simulink model "loader_est"  (R2025b)
settings: Solver=FixedStepAuto  StartTime=0.0  StopTime=26  FixedStep=0.001  RelTol=1e-3
undefined symbols (not defined in the file or in its folder): m_arm, m_bucket, m_load, X, Y, Z
libraries: sm_lib x31, nesl_utility x10, simulink x1
(part 2 of 2)

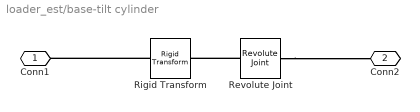
== system loader_est/base-tilt cylinder ==
  Revolute Joint : sm_lib/Joints/Revolute Joint  JointMode=Normal  CompositeWrenchDir=FollowerOnBase  CompositeWrenchFrame=BaseFrame  SenseConstraintForce=off  SenseConstraintTorque=off  SenseTotalForce=off  SenseTotalTorque=off  PositionTargetSpecify=off  PositionTargetPriority=High  PositionTargetValue=0  PositionTargetValueUnits=deg  VelocityTargetSpecify=off  VelocityTargetPriority=High  VelocityTargetValue=0  VelocityTargetValueUnits=deg/s  EquilibriumPosition=0  EquilibriumPositionUnits=deg  SpringStiffness=0  SpringStiffnessUnits=N*m/deg  DampingCoefficient=0  DampingCoefficientUnits=N*m/(deg/s)  LowerLimitSpecify=off  LowerLimitBound=-90  LowerLimitBoundUnits=deg  LowerLimitStiffness=1e4  LowerLimitStiffnessUnits=N*m/deg  LowerLimitDamping=10  LowerLimitDampingUnits=N*m/(deg/s)  LowerLimitTransitionRegionWidth=0.1  LowerLimitTransitionRegionWidthUnits=deg  UpperLimitSpecify=off  UpperLimitBound=90  UpperLimitBoundUnits=deg  UpperLimitStiffness=1e4  UpperLimitStiffnessUnits=N*m/deg  UpperLimitDamping=10  UpperLimitDampingUnits=N*m/(deg/s)  UpperLimitTransitionRegionWidth=0.1  UpperLimitTransitionRegionWidthUnits=deg  TorqueActuationMode=NoTorque  MotionActuationMode=ComputedMotion  SensePosition=off  SenseVelocity=off  SenseAcceleration=off  SenseTorqueForce=off  SenseLowerLimitTorqueForce=off  SenseUpperLimitTorqueForce=off
  Rigid Transform : sm_lib/Frames and Transforms/Rigid Transform  RotationMethod=RotationSequence  FollAlignAxisA=+X  BaseAlignAxisA=+Y  FollAlignAxisB=+Y  BaseAlignAxisB=+Z  RotationStandardAxis=+Z  RotationAngle=0  RotationAngleUnits=deg  RotationArbitraryAxis=[0 0 1]  RotationSequenceAxes=FollowerAxes  RotationSequence=XYX  RotationSequenceAngles=[90 180 0]  RotationSequenceAnglesUnits=deg  RotationMatrix=[1 0 0;0 1 0;0 0 1]  Quaternion=[1 0 0 0]  TranslationMethod=Cartesian  TranslationCartesianOffset=[35 0 -7]  TranslationCartesianOffsetUnits=cm  TranslationStandardAxis=+Z  TranslationStandardOffset=0  TranslationStandardOffsetUnits=m  TranslationROffset=0  TranslationROffsetUnits=m  TranslationThetaOffset=0  TranslationThetaOffsetUnits=deg  TranslationZOffset=0  TranslationZOffsetUnits=m
  Conn1 : PMIOPort  Side=Left
  Conn2 : PMIOPort  Port=2  Side=Right
  connections:
  Revolute Joint/LConn1 -- Rigid Transform/RConn1
  Revolute Joint/RConn1 -- Conn2/RConn1
  Rigid Transform/LConn1 -- Conn1/RConn1

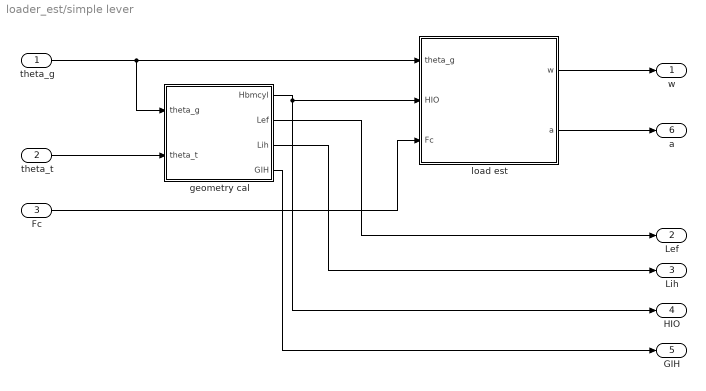
== system loader_est/simple lever  ==
  theta_g : Inport
  theta_t : Inport  Port=2
  Fc : Inport  Port=3
  geometry cal : MATLAB Function  TreatAsAtomicUnit=on
  load est : MATLAB Function  TreatAsAtomicUnit=on
  w : Outport
  Lef : Outport  Port=2
  Lih : Outport  Port=3
  HIO : Outport  Port=4
  GIH : Outport  Port=5
  a : Outport  Port=6
  wires:
  geometry cal/1(Hbmcyl) -> HIO/1, load est/2(HIO)
  Fc/1 -> load est/3(Fc)
  geometry cal/2(Lef) -> Lef/1
  geometry cal/3(Lih) -> Lih/1
  theta_g/1 -> geometry cal/1(theta_g), load est/1(theta_g)
  load est/1(w) -> w/1
  theta_t/1 -> geometry cal/2(theta_t)
  geometry cal/4(GIH) -> GIH/1
  load est/2(a) -> a/1

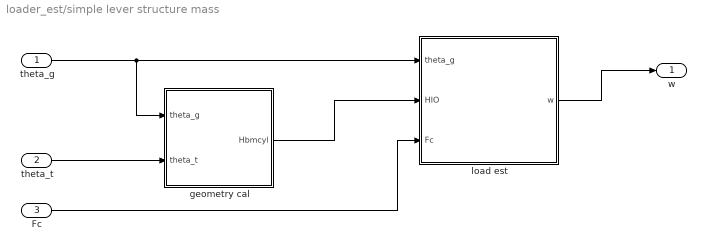
== system loader_est/simple lever structure mass ==
  theta_g : Inport
  theta_t : Inport  Port=2
  Fc : Inport  Port=3
  geometry cal : MATLAB Function  TreatAsAtomicUnit=on
  load est : MATLAB Function  TreatAsAtomicUnit=on
  w : Outport
  wires:
  geometry cal/1(Hbmcyl) -> load est/2(HIO)
  Fc/1 -> load est/3(Fc)
  theta_g/1 -> geometry cal/1(theta_g), load est/1(theta_g)
  load est/1(w) -> w/1
  theta_t/1 -> geometry cal/2(theta_t)

== matlab function loader_est/simple lever /load est ==
  data: theta_g input; w output; HIO input; Fc input; a output
function [w,a] = fcn(theta_g, HIO, Fc)
Lgh = 1630;
Lag = 3929.4;
w = ((Fc*Lgh/Lag) * (sind(HIO) - cosd(HIO)*tand(theta_g)))/9.81;
a = sind(HIO) - cosd(HIO)*tand(theta_g);

== matlab function loader_est/MATLAB Function ==
  data: theta_g input; g output; theta_t input; t output
function [g,t]= fcn(theta_g, theta_t)

g_offset = 39.35;
t_offset = -74.89;

g = theta_g + g_offset;
t = theta_t + t_offset;

== matlab function loader_est/simple lever /geometry cal ==
  data: theta_g input; Hbmcyl output; theta_t input; Lef output; Lih output; GIH output
function [Hbmcyl,Lef,Lih,GIH] = fcn(theta_g, theta_t)

Ldg = 2494.4; 
Lfg = 356.9;
Lde = 926.3;
LgiX = -13.5*10;
LgiY = -64*10;
Lgi = sqrt(LgiY^2 + LgiX^2); % 654.0833
Lgh = 1630;
DGA = 16.38;
LfgX = 350;
LfgY = 70;
FGO = atand(LfgY/LfgX); % 11.3099
DEC = 180-162.65;       % 17.3500
IGO = 180 - atand(LgiY/LgiX); % IGO = 101.9112

FGD = FGO + theta_g + DGA;
Ldf = sqrt(Lfg^2 + Ldg^2 - 2*Lfg*Ldg*cosd(FGD));

DEF = theta_t + DEC;
EFD = asind(Lde*sind(DEF) / Ldf);
EDF = 180 - EFD - DEF;

% tilt prismatic length
Lef = Lde*sind(EDF) / sind(EFD);

% lift prismatic length
Lih = sqrt(Lgh^2 + Lgi^2 - 2*Lgh*Lgi*cosd(theta_g + IGO));
GIH = asind((Lgh/Lih) * sind(theta_g + IGO));
Hbmcyl = (180 - IGO) - GIH;

== matlab function loader_est/MATLAB Function1 ==
  data: theta_g input; w output; f output; theta_t input; Fc input; theta_i output
function [w,f,theta_i] = fcn(theta_g, theta_t, Fc)

Ldg = 2494.4; 
Lfg = 356.9;
LfgX = 350;
LfgY = 70;
Lag = 3929.4;
Lde = 926.3;
Lad = 1689.5;
Lcd = 1133.2;
Lbc = 984.4;
Lab = 454.8;
LgiX = -13.5*10;
LgiY = -64*10;
Lgi = sqrt(LgiY^2 + LgiX^2); % 654.0833
Lgh = 1630;

DGA = 16.38;
FGO = atand(LfgY/LfgX); % 11.3099
theta_d = 180-148.55 ;  % 31.4500
DEC = 180-162.65  ;     % 17.3500
IGO = 180 - atand(LgiY/LgiX); % IGO = 101.9112

% *eq 15
FGD = FGO + theta_g + DGA;
Ldf = sqrt(Lfg^2 + Ldg^2 - 2*Lfg*Ldg*cosd(FGD));

% add
DEF = theta_t + DEC;
EFD = asind(Lde*sind(DEF) / Ldf);
EDF = 180 - EFD - DEF;
% tilt prismatic length
Lef = Lde*sind(EDF) / sind(EFD);

% eq 17
a3 = Ldg*sind(theta_g + DGA) - LfgY;
a4 = Ldg*cosd(theta_g + DGA) - LfgX;
a5 = Ldf^2 + Lef^2 - Lde^2;
a6 = 2*Ldf*Lef;
theta_f = atand(a3/a4) + acosd(a5/a6);

theta_e = -(180 - DEC - theta_t);

% eq 19
a9 = Lad^2 + Ldg^2 - Lag^2;
a10 = 2*Lad*Ldg;
ADC = acosd(a9/a10) + EFD - 180 - theta_d;

% eq 20
Lac = sqrt(Lad^2 + Lcd^2 - 2*Lad*Lcd*cosd(ADC));

% eq 21
a13 = Lac^2 + Lbc^2 - Lab^2;
a14 = 2*Lac*Lbc;
a15 = Lcd^2 + Lac^2 - Lad^2;
a16 = 2*Lcd*Lac;
theta_c = 180 + acosd(a13/a14) - acosd(a15/a16);

% eq 22
a17 = Lab^2 + Lbc^2 - Lac^2;
a18 = 2*Lab*Lbc;
theta_b = acosd(a17/a18) - 180;

% lift prismatic length
Lih = sqrt(Lgh^2 + Lgi^2 - 2*Lgh*Lgi*cosd(theta_g + IGO));

GIH = asind((Lgh/Lih) * sind(theta_g + IGO));

% *eq 14
Hbmcyl = (180- IGO) - GIH;
theta_i = 180 - (IGO + Hbmcyl) ;

% *eq 7
LloadG = 500;
HloadG = 0;
a21 = theta_g + theta_c + theta_e - theta_b + 180 - HloadG;
a = LloadG*cosd(a21);

% eq 8
b = -Lab*sind(theta_b);
% eq 9 
c = Lcd*sind(theta_c);
% eq 10
d = -Lde*sind(theta_e);
% eq 11
e = Lfg*sind(180 - theta_f + FGO);
% eq 12
f = Lgi*sind(theta_i);
% eq 13
Lw = Lag*cosd(theta_g) + a;


w = (f*Fc / (Lw - a*c*e*b^(-1)*d^(-1)))/9.81;

== matlab function loader_est/simple lever structure mass/geometry cal ==
  data: theta_g input; Hbmcyl output; theta_t input
function Hbmcyl = fcn(theta_g, theta_t)

Ldg = 2494.4; 
Lfg = 356.9;
Lde = 926.3;
LgiX = -13.5*10;
LgiY = -64*10;
Lgi = sqrt(LgiY^2 + LgiX^2); % 654.0833
Lgh = 1630;
DGA = 16.38;
LfgX = 350;
LfgY = 70;
FGO = atand(LfgY/LfgX); % 11.3099
DEC = 180-162.65;       % 17.3500
IGO = 180 - atand(LgiY/LgiX); % IGO = 101.9112

FGD = FGO + theta_g + DGA;
Ldf = sqrt(Lfg^2 + Ldg^2 - 2*Lfg*Ldg*cosd(FGD));

DEF = theta_t + DEC;
EFD = asind(Lde*sind(DEF) / Ldf);
EDF = 180 - EFD - DEF;

% tilt prismatic length
Lef = Lde*sind(EDF) / sind(EFD);

% lift prismatic length
Lih = sqrt(Lgh^2 + Lgi^2 - 2*Lgh*Lgi*cosd(theta_g + IGO));
GIH = asind((Lgh/Lih) * sind(theta_g + IGO));
Hbmcyl = (180 - IGO) - GIH;

== matlab function loader_est/simple lever structure mass/load est ==
  data: theta_g input; w output; HIO input; Fc input
function w = fcn(theta_g, HIO, Fc)
Lgh = 1630;
Lag = 3929.4;
a = sind(HIO) - cosd(HIO)*tand(theta_g);
k = 
b = 
w = ((Fc*Lgh/Lag) * a)/9.81;
